simulink model "pend_2020a"  (R2020a)
settings: Solver=VariableStepAuto  StartTime=0.0  StopTime=10.0  RelTol=1e-3
values from neighbouring files (symbols this model uses):
  g = 9.8    [param_pend.m]
  l = 1.0    (= 1)    [param_pend.m]
settings Model: Creator=fukao  LastModifiedBy=fukao
settings DebuggingCC: SFMachineParentedDataDiag=error

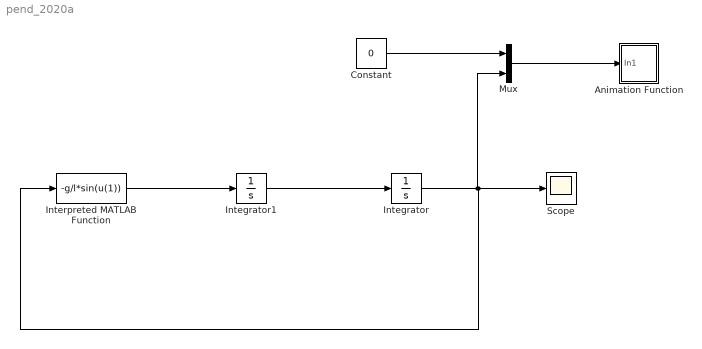
== system pend_2020a ==
  Animation Function : Subsystem  mask(Animation Block){ts=0.05}
      mask prompts: ts "Sample time:"
      mask Display: plot([.1,.9],[.9,.9],[.5,.2],[.9,.25],[.475,.475,.525,.525,.475],[.875,.925,.925,.875,.875])
  Constant : Constant  Value=0
  Integrator : Integrator  InitialCondition=0.5
  Integrator1 : Integrator
  Interpreted MATLAB Function : MATLABFcn  MATLABFcn=-g/l*sin(u(1))
  Mux : Mux  Inputs=2
  Scope : Scope
  wires:
  Integrator/1 -> Mux/2, Interpreted MATLAB Function/1, Scope/1
  Integrator1/1 -> Integrator/1
  Interpreted MATLAB Function/1 -> Integrator1/1
  Mux/1 -> Animation Function/1(In1)
  Constant/1 -> Mux/1

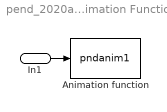
== system pend_2020a/Animation Function ==
  In1 : Inport
  Animation function : S-Function  FunctionName=pndanim1  Parameters=ts  SFunctionDeploymentMode=off  EnableBusSupport=off
      settings: DeleteFcn=if ~isempty(findobj('type','figure','name','simppend Animation'));close('simppend Animation'); end;
  wires:
  In1/1 -> Animation function/1
